simulink model "Caracterizacion"  (R2016b)
settings: Solver=FixedStepDiscrete  StartTime=0.0  StopTime=20  FixedStep=0.05  RelTol=1e-3  EnableMultiTasking=on
libraries: arduinolib x8
settings Model: ExtModeTrigDuration=2  Creator=Julian  LastModifiedBy=Julian
settings OptimizationCC: MaxStackSize=64
settings DebuggingCC: ParameterTunabilityLossMsg=error
settings HardwareCC: ProdBitPerInt=16  ProdBitPerPointer=16  ProdBitPerSizeT=16  ProdBitPerPtrDiffT=16  ProdLargestAtomicFloat=None  ProdWordSize=8  ProdHWDeviceType=Atmel->AVR
settings RTWCC: SystemTargetFile=ert.tlc  HardwareBoard=Arduino Mega 2560  TLCOptions=-aInlineSetEventsForThisBaseRateFcn=TLC_FALSE -aSuppressMultiTaskScheduler=TLC_FALSE -aRateBasedStepFcn=1  TemplateMakefile=ert_default_tmf  Description=Embedded Coder  GenerateReport=on  Toolchain=Arduino AVR  BuildConfiguration=Faster Runs  IncludeHyperlinkInReport=on  LaunchReport=on  GenerateTraceInfo=on  GenerateTraceReport=on  GenerateTraceReportSl=on  GenerateTraceReportSf=on  GenerateTraceReportEml=on
settings CodeAppCC: ForceParamTrailComments=on  IgnoreCustomStorageClasses=off  OperatorAnnotations=on  SimulinkDataObjDesc=on  SFDataObjDesc=on  MATLABFcnDesc=on  InsertBlockDesc=on  MATLABSourceComments=on
settings ERTTargetCC: SupportContinuousTime=on  SupportVariableSizeSignals=on

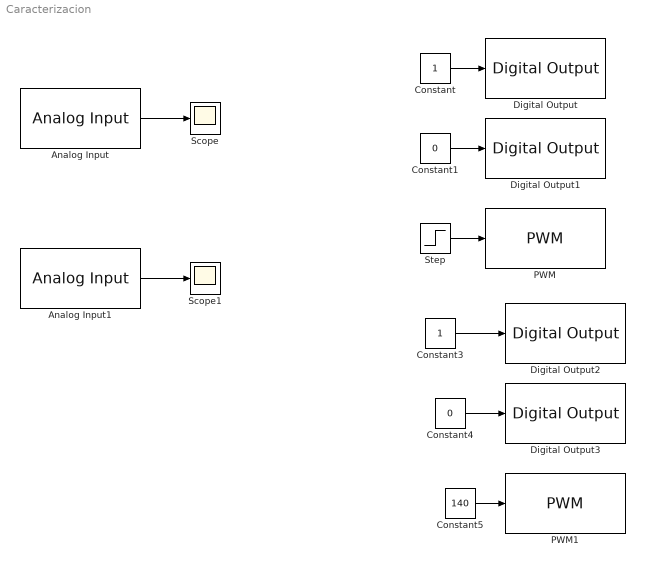
== system Caracterizacion ==
  Analog Input : arduinolib/Analog Input  pinNumber=0  sampleTime=0.1  blockPlatform=arduino
  Analog Input1 : arduinolib/Analog Input  pinNumber=1  sampleTime=0.1  blockPlatform=arduino
  Constant : Constant
  Constant1 : Constant  Value=0
  Constant3 : Constant
  Constant4 : Constant  Value=0
  Constant5 : Constant  Value=140
  Digital Output : arduinolib/Digital Output  pinNumber=2  blockPlatform=arduino
  Digital Output1 : arduinolib/Digital Output  pinNumber=3  blockPlatform=arduino
  Digital Output2 : arduinolib/Digital Output  pinNumber=7  blockPlatform=arduino
  Digital Output3 : arduinolib/Digital Output  pinNumber=8  blockPlatform=arduino
  PWM : arduinolib/PWM  pinNumber=4  blockPlatform=arduino
  PWM1 : arduinolib/PWM  pinNumber=9  blockPlatform=arduino
  Scope : Scope
  Scope1 : Scope
  Step : Step  Time=2  Before=30  After=0  SampleTime=0
  wires:
  Analog Input/1 -> Scope/1
  Analog Input1/1 -> Scope1/1
  Constant/1 -> Digital Output/1
  Constant1/1 -> Digital Output1/1
  Constant3/1 -> Digital Output2/1
  Constant4/1 -> Digital Output3/1
  Constant5/1 -> PWM1/1
  Step/1 -> PWM/1
